simulink model "powerwindow03"  (Simulink 10.0)
settings: Solver=ode23tb  StartTime=0.0  StopTime=inf  FixedStep=1e-4  RelTol=1e-2  EnableMultiTasking=on
libraries: mblibv1 x19, powerlib x15, simulink x4, vrlib x1
(part 2 of 2)

== stateflow chart power_window_control_system/control ==
  settings: executeAtInitialization=1
  state safe
    state driverNeutral
      entry:
      moveUp = 0;
      moveDown = 0;
      state passengerneutral
        entry:
        moveUp = 0;
        moveDown = 0;
      state passengerDown
        entry: moveDown = 1;
        exit: moveDown = 0;
        state iniPassengerDown
        state passengerDown
        state autoPassengerDown
        iniPassengerDown -> (junction 41) : after(100,ticks)
        (junction 41) -> autoPassengerDown [order 1] : [passenger[1]]
        (junction 41) -> safe.driverNeutral.passengerDown.passengerDown [order 2]
      state passengerUp
        entry: moveUp = 1;
        exit: moveUp = 0;
        state iniPassengerUp
        state PassengerUp
        state autoPassengerUp
        iniPassengerUp -> (junction 45) : after(100,ticks)
        (junction 45) -> PassengerUp [order 2]
        (junction 45) -> autoPassengerUp [order 1] : [passenger[1]]
      (default) -> passengerneutral
      passengerneutral -> iniPassengerUp [order 1] : [passenger[2]]
      passengerneutral -> iniPassengerDown [order 2] : [passenger[3]]
      safe.driverNeutral.passengerDown.passengerDown -> passengerneutral : [passenger[1]]
      safe.driverNeutral.passengerDown -> passengerneutral [order 1] : [endstop]
      PassengerUp -> passengerneutral : [passenger[1]]
      passengerUp -> passengerneutral [order 2] : [endstop]
      safe.driverNeutral.passengerDown -> PassengerUp [order 2] : [passenger[2]]
      passengerUp -> safe.driverNeutral.passengerDown.passengerDown [order 1] : [passenger[3]]
    state driverDown
      entry: moveDown = 1;
      exit: moveDown = 0;
      state iniDriverDown
      state autoDriverDown
      state DriverDown
      iniDriverDown -> (junction 49) : after(100,ticks)
      (junction 49) -> autoDriverDown [order 1] : [driver[1]]
      (junction 49) -> DriverDown [order 2]
    state driverUp
      entry: moveUp = 1;
      exit: moveUp = 0;
      state iniDriverUp
      state DriverUp
      state autoDriverUp
      iniDriverUp -> (junction 53) : after(100,ticks)
      (junction 53) -> DriverUp [order 2]
      (junction 53) -> autoDriverUp [order 1] : [driver[1]]
    (default) -> driverNeutral
    driverNeutral -> iniDriverDown [order 2] : [driver[3]]
    DriverDown -> driverNeutral : [driver[1]]
    driverDown -> driverNeutral [order 1] : [endstop]
    DriverUp -> driverNeutral : [driver[1]]
    driverUp -> driverNeutral [order 2] : [endstop]
    driverNeutral -> iniDriverUp [order 1] : [driver[2]]
    driverDown -> DriverUp [order 2] : [driver[2]]
    driverUp -> DriverDown [order 1] : [driver[3]]
  state emergencyDown
    entry:
    moveUp = 0;
    moveDown = 1;
  emergencyDown -> passengerneutral : [endstop | after(100,ticks)]
  (default) -> safe
  safe -> emergencyDown : [obstacle]
  data: moveUp output double; moveDown output double; endstop input boolean; obstacle input boolean; driver input boolean size=3; passenger input boolean size=3
  events: ticks input EITHER_EDGE_EVENT

== stateflow chart power_window_control_system/detect_obstacle_endstop/detect_obstacle/delay_detection ==
  settings: executeAtInitialization=1
  state off
  state hold
  state detect
  (default) -> off
  off -> hold : [move_up]
  detect -> off : [~move_up]
  hold -> off [order 2] : [~move_up]
  hold -> detect [order 1] : [after(100,ticks)]
  data: detect output unknown; move_up input boolean
  events: ticks input EITHER_EDGE_EVENT
